simulink model "verify_alfa_window_in_mdl"  (R2018b)
settings: Solver=VariableStepDiscrete  StartTime=6*3600  StopTime=18*3600  MaxStep=1  RelTol=1e-3  EnableMultiTasking=on
libraries: carnot x5
settings Model: Creator=drhf  LastModifiedBy=drhf
settings DataIOCC: SaveFormat=Array  SignalLoggingSaveFormat=ModelDataLogs
settings OptimizationCC: ExpressionDepthLimit=2147483647  LifeSpan=inf
settings DebuggingCC: UnderspecifiedInitializationDetection=Classic  MergeDetectMultiDrivingBlocksExec=none  SolverPrmCheckMsg=warning  StateNameClashWarn=warning  SFUnexpectedBacktrackingDiag=warning  SFNoUnconditionalDefaultTransitionDiag=warning  SFExecutionAtInitializationDiag=none
settings HardwareCC: ProdBitPerPointer=32  ProdBitPerSizeT=32  ProdBitPerPtrDiffT=32  ProdLargestAtomicFloat=None  ProdIntDivRoundTo=Undefined  ProdEndianess=Unspecified  ProdWordSize=32  ProdHWDeviceType=32-bit Generic
settings ModelReferenceCC: PropagateSignalLabelsOutOfModel=off
settings SFSimCC: SimUseLocalCustomCode=off
settings RTWCC: RTWUseLocalCustomCode=off
settings CodeAppCC: StateflowObjectComments=on
settings GRTTargetCC: TargetLangStandard=C89/C90 (ANSI)  GeneratePreprocessorConditionals=Disable all  CombineOutputUpdateFcns=off  GRTInterface=on
settings ConfigComp: CovMetricSettings=dw  CovHtmlReporting=on  CovSaveCumulativeToWorkspaceVar=on  CovSaveSingleToWorkspaceVar=on  CovExternalEMLEnable=off

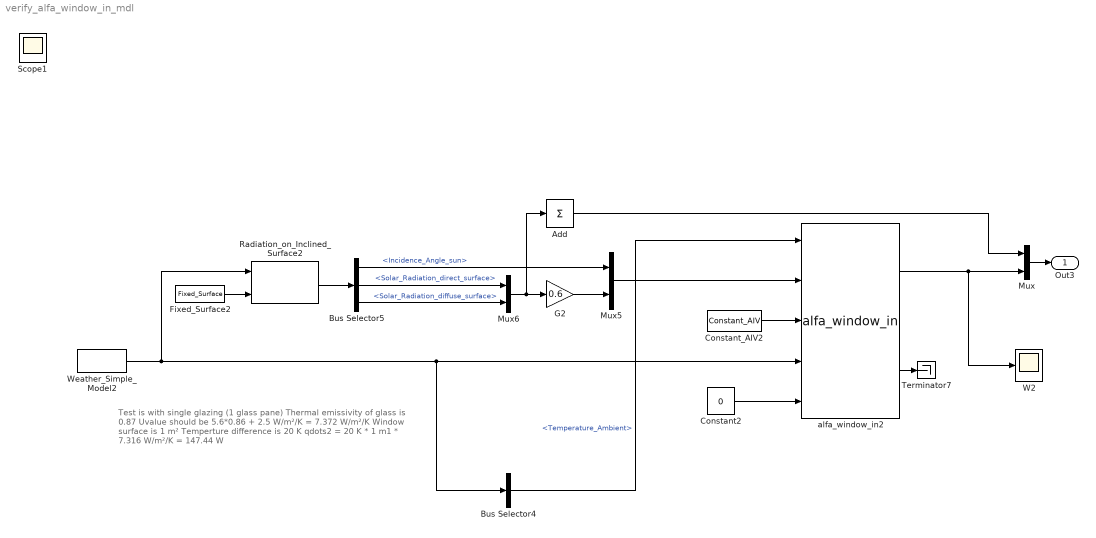
== system verify_alfa_window_in_mdl ==
  note: Test is with single glazing (1 glass pane)
      | Thermal emissivity of glass is 0.87
      | Uvalue should be 5.6*0.86 + 2.5 W/m²/K = 7.372 W/m²/K
      | Window surface is 1 m²
      | Temperture difference is 20 K
      | qdots2 = 20 K * 1 m1 * 7.316 W/m²/K = 147.44 W
  Add : Sum  Inputs=1
  Bus Selector4 : BusSelector  OutputSignals=Temperature_Ambient
  Bus Selector5 : BusSelector  OutputSignals=Incidence_Angle_sun,Solar_Radiation_direct_surface,Solar_Radiation_diffuse_surface
  Constant2 : Constant  Value=0
  Constant_AIV2 : carnot/Source/Ventilation/Constant_AIV  Tsens=20  Tcon=20  Trad=20  mw=0.012  mco=0.01  rhoair=1.2  cpair=1004  pair=100000  nair=0.5
      settings: SourceProductName=Carnot
  Fixed_Surface2 : carnot/Weather/Fixed_Surface  colangle=90  colazi=0  colrot=0
      settings: SourceProductName=Carnot
  G2 : Gain  Gain=0.6
  Mux : Mux  Inputs=2
  Mux5 : Mux  Inputs=2
  Mux6 : Mux  Inputs=2
  Radiation_on_Inclined_Surface2 : carnot/Weather/Radiation_on_Inclined_Surface  sky=Perez 1990  reflect=0.2
      settings: SourceProductName=Carnot
  Terminator7 : Terminator
  W2 : Scope
  Weather_Simple_Model2 : carnot/Weather/Weather_Simple_Model  Ibn=900  Idg=100  tamb=0  deltaTsky=0  rh=50  precip="10e-3/24/3600           % 10 mm in 24 h"  cloud=0.125  p=1013e2  vw=0  wdir=270  lat=60  colangle=0  colazi=0  colrot=0
      settings: SourceProductName=Carnot
  alfa_window_in2 : carnot/Basic/Heat_Transfer/alfa_window_in  type_glazing=double glazing normal  gvalue=0.8  tauzero=0.9  emission_in=0.87  wallsurface=1  frame=0  numlayer=1  shad_type=No shading  tau_shad=0.01  bli_a=0.05  bli_b=1  bli_c=0.05  bli_d=0.05  bli_alpha=90  bli_refl=0.2
      settings: SourceProductName=Carnot
  Out3 : Outport
  Scope1 : Scope
  wires:
  alfa_window_in2/2 -> Terminator7/1
  alfa_window_in2/1 -> W2/1, Mux/2
  Constant_AIV2/1 -> alfa_window_in2/3
  Weather_Simple_Model2/1 -> Radiation_on_Inclined_Surface2/1, Bus Selector4/1, alfa_window_in2/4
  Constant2/1 -> alfa_window_in2/5
  Bus Selector4/1 -> alfa_window_in2/1  "<Temperature_Ambient>"
  Radiation_on_Inclined_Surface2/1 -> Bus Selector5/1
  Bus Selector5/2 -> Mux6/1  "<Solar_Radiation_direct_surface>"
  Bus Selector5/1 -> Mux5/1  "<Incidence_Angle_sun>"
  Mux5/1 -> alfa_window_in2/2
  G2/1 -> Mux5/2
  Bus Selector5/3 -> Mux6/2  "<Solar_Radiation_diffuse_surface>"
  Fixed_Surface2/1 -> Radiation_on_Inclined_Surface2/2
  Mux6/1 -> Add/1, G2/1
  Mux/1 -> Out3/1
  Add/1 -> Mux/1
